simulink model "projectsimulink"  (R2021a)
settings: Solver=VariableStepAuto  StartTime=0.0  StopTime=10000  RelTol=1e-3
libraries: commrandsrc3 x1, spspowerguiLib x1
settings Model: Creator=ziada  LastModifiedBy=ziada
settings OptimizationCC: DefaultParameterBehavior=Inlined  EnhancedBackFolding=on  PassReuseOutputArgsAs=Individual arguments  ZeroExternalMemoryAtStartup=off  ZeroInternalMemoryAtStartup=off  OptimizeBlockOrder=speed  DifferentSizesBufferReuse=on  OptimizationCustomize=off  EfficientTunableParamExpr=on
settings DebuggingCC: ParameterTunabilityLossMsg=error
settings SFSimCC: MATLABDynamicMemAlloc=off
settings RTWCC: SystemTargetFile=ert.tlc  TemplateMakefile=ert_default_tmf
settings CodeAppCC: ForceParamTrailComments=on  IgnoreCustomStorageClasses=off  OperatorAnnotations=on  SimulinkDataObjDesc=on  SFDataObjDesc=on  InsertBlockDesc=on
settings ERTTargetCC: TargetLangStandard=C99 (ISO)  GenerateSampleERTMain=on  InlinedParameterPlacement=NonHierarchical  ERTCustomFileTemplate=example_file_process.tlc

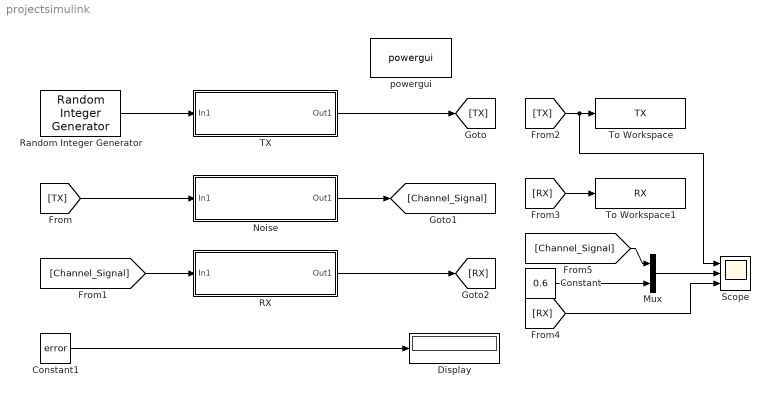
== system projectsimulink ==
  Constant : Constant  Value=0.6
  Constant1 : Constant  Value=error
  Display : Display
  Mux : Mux  Inputs=2
  Noise : Subsystem
  RX : Subsystem
  Random Integer Generator : commrandsrc3/Random Integer Generator  SetSize=2  SeedSource=Auto  Seed=3  SampleTime=1  SamplesPerFrame=1  OutputDataType=boolean  SimulateUsing=Interpreted execution
  Scope : Scope  NumInputPorts=3
  TX : Subsystem
  To Workspace : ToWorkspace  VariableName=TX  SampleTime=-1
      settings: Save2DSignal=2-D array (concatenate along first dimension)
  To Workspace1 : ToWorkspace  VariableName=RX  SampleTime=-1
      settings: Save2DSignal=2-D array (concatenate along first dimension)
  powergui : spspowerguiLib/powergui  Priority=1  SimulationMode=Continuous  SampleTime=50e-6  frequency=60  Iterations=50  frequencyindice=60  Pbase=100e6  ErrMax=1e-4  UnitsV=kV  UnitsW=MW  buscounter=0  FunctionMessages=off  echomessages=off  EnableUseOfTLC=off  CurrentSourceSwitches=off  DisableSnubberDevices=off  DisableRonSwitches=off  DisableVfSwitches=off  DisplayEquations=off  AutomaticDiscreteSolvers=off  SolverType=Tustin/Backward Euler (TBE)  Interpol=off  ExternalGateDelay=off  methode=off  Ts=100  x0status=blocks  SPID=on  SwTol=0  HookPort=off  NonlinearTolerance=1e-4  nMaxIteration=100  ContinueOnMaxIteration=off  RestoreLinks=warning  ResistiveCurrentMeasurement=off  Frange=[0:2:500]  Ylog=off  Xlog=on  ShowGrid=off  save=off  variable=ZData  structure=0  ZoomFFT=off  StartTime=0.0  cycles=1  DisplayStyle=1  fundamental=60  FreqAxis=off  MaxFrequency=1000  frequencyindicesteady=1  RmsSteady=1  display=off
  wires:
  Random Integer Generator/1 -> TX/1(In1)
  TX/1(Out1) -> [TX]
  [TX] -> Noise/1(In1)
  Noise/1(Out1) -> [Channel_Signal]
  [Channel_Signal] -> RX/1(In1)
  RX/1(Out1) -> [RX]
  [RX] -> To Workspace1/1
  [TX] -> Scope/1, To Workspace/1
  [RX] -> Scope/3
  [Channel_Signal] -> Mux/1
  Constant/1 -> Mux/2
  Mux/1 -> Scope/2
  Constant1/1 -> Display/1

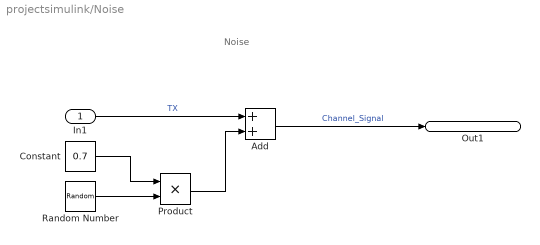
== system projectsimulink/Noise ==
  note: Noise
  In1 : Inport
  Add : Sum
  Constant : Constant  Value=0.7
  Product : Product
  Random Number : RandomNumber  SampleTime=1
  Out1 : Outport
  wires:
  Product/1 -> Add/2
  In1/1 -> Add/1  "TX"
  Constant/1 -> Product/1
  Add/1 -> Out1/1  "Channel_Signal"
  Random Number/1 -> Product/2

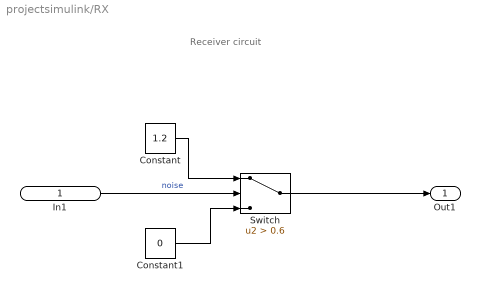
== system projectsimulink/RX ==
  note: Receiver circuit
  In1 : Inport
  Constant : Constant  Value=1.2
  Constant1 : Constant  Value=0
  Switch : Switch  Criteria=u2 > Threshold  Threshold=0.6
  Out1 : Outport
  wires:
  In1/1 -> Switch/2  "noise"
  Constant/1 -> Switch/1
  Constant1/1 -> Switch/3
  Switch/1 -> Out1/1

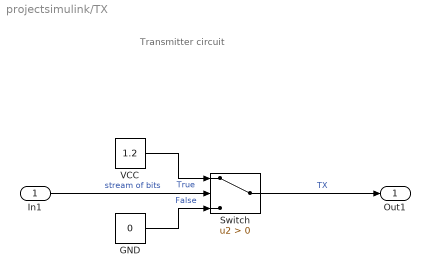
== system projectsimulink/TX ==
  note: Transmitter circuit
  In1 : Inport
  GND : Constant  Value=0
  Switch : Switch  Criteria=u2 > Threshold
  VCC : Constant  Value=1.2
  Out1 : Outport
  wires:
  VCC/1 -> Switch/1  "True"
  GND/1 -> Switch/3  "False"
  Switch/1 -> Out1/1  "TX"
  In1/1 -> Switch/2  "stream of bits"
